simulink model "BMS_MainStateMachine_COM_Harness_SIL"  (R2022b)
settings: configuration reference "BMS_Sw_CodeGenConfig" (kept outside this file)
model workspace (MAT data in the model file):
  BATT.Manufacturer = 'Panasonic'
  BATT.Chemistry = 'Lithium Ion'
  BATT.Model = 'UR18650ZTA'
  BATT.Diameter = 18.2399997711
  BATT.Length = 65.0999984741
  BATT.CycleLife = 500
  BATT.Package.Ns_Module = 1
  BATT.Package.NumModules = 3
  BATT.Capacity.Rate = 2.84999990463
  BATT.Capacity.Min = 2.90000009537
  BATT.Capacity.Max = 3.09999990463
  BATT.Capacity.MaxQ = 3.30460000038
  BATT.Capacity.Type = 3
  BATT.Res.R0 = 0.0113329999149
  BATT.Res.R1 = 0.00999999977648
  BATT.Res.C1 = 0.00300000002608
  BATT.Res.R0_EOL = 0.0142999999225
  BATT.Res.lambda = 1.06599998474
  BATT.Voltage.Nominal = 3.70000004768
  BATT.Voltage.NominalVolt = 3.40000009537
  BATT.Voltage.Cut_off = 3
  BATT.Voltage.Init_Dchrg = 3.38000011444
  BATT.Voltage.Full_Dchrg = 4.19999980927
  BATT.Voltage.Max_Chrg = 4.34999990463
  BATT.Voltage.Over = 4.40000009537
  BATT.Voltage.Under = 3
  BATT.Voltage.threshold = 0.5
  BATT.Voltage.V_LUT = [3 3.09999990463 3.20000004768 3.29999995232 3.40000009537 3.5 3.59999990463 3.70000004768 3.79999995232 3.90000009537 4 4.09999990463 4.19999980927]
  BATT.Temperature.Max = 50
  BATT.Temperature.Min = -20
  BATT.Temperature.Nominal = 20
  BATT.Temperature.dQ_dt = 0.00499999988824
  BATT.Temperature.T_LUT = [-20 -15 -10 -5 0 5 10 15 20 25 30 35 40 45 50]
  BATT.Temperature.derate_Fact = [0.598999977112 0.69580000639 0.769999980927 0.824599981308 0.870000004768 0.912999987602 0.949999988079 0.981000006199 1 1.00499999523 1.00999999046 1.01800000668 1.02999997139 1.05700004101 1.10000002384]
  BATT.Current.Dchrg = 6
  BATT.Current.Chrg = 1.45000004768
  BATT.Current.Chrgfast = 2.5
  BATT.Current.ChrgSafe = 0.0579999983311
  BATT.Current.Overthreshold = 0.20000000298
  BATT.Current.threshold = 0.00999999977648
  BATT.Current.CV_Gain = 20
  BATT.SoC.SoC0 = 50
  BATT.SoC.max = 100
  BATT.SoC.min = 0
  BATT.SoC.alpha = 0.25
  BATT.SoC.Values = [0 10 20 30 40 50 60 70 80 90 100]
  BATT.SoC.iter = 10
  BATT.SoC.TableData = [20 30 40 55 70 85 90 100 100 100 100 100 ... (195 elements, 13x15)]
  BATT.Balancing.Mode : BMS_BalMode_Enum (value not decoded)
  BATT.Balancing.ThresholdOn = 0.0250000003725
  BATT.Balancing.ThresholdOff = 0.00999999977648
  BATT.Balancing.BalWaitOff = 5
  BATT.Balancing.BalWaitOn = 10
  BATT.Balancing.Freq = 1000
  BATT.Balancing.Duty = 0.449999988079
  ChrgBit = Simulink.Parameter
  ChrgBit.Value = 0
  ChrgBit.Description = 'charger Fault Bit'
  ChrgBit.DataType = 'uint8'
  ChrgBit.Complexity = 'real'
  ChrgBit.Dimensions = [1 1]
  CntTime = Simulink.Parameter
  CntTime.Value = 500
  CntTime.Description = 'Conector waiting Time'
  CntTime.DataType = 'uint16'
  CntTime.Complexity = 'real'
  CntTime.Dimensions = [1 1]
  CntTimeout = Simulink.Parameter
  CntTimeout.Value = 5000
  CntTimeout.Description = 'Conector Timeout'
  CntTimeout.DataType = 'uint16'
  CntTimeout.Complexity = 'real'
  CntTimeout.Dimensions = [1 1]
  CurrTimeout = Simulink.Parameter
  CurrTimeout.Value = 1000
  CurrTimeout.Description = 'Over Current Timeout'
  CurrTimeout.DataType = 'uint16'
  CurrTimeout.Complexity = 'real'
  CurrTimeout.Dimensions = [1 1]
  FaultResetTime = Simulink.Parameter
  FaultResetTime.Value = 5000
  FaultResetTime.Description = 'Fault Reset waiting Time'
  FaultResetTime.DataType = 'uint16'
  FaultResetTime.Complexity = 'real'
  FaultResetTime.Dimensions = [1 1]
  HighTempBit = Simulink.Parameter
  HighTempBit.Value = 4
  HighTempBit.Description = 'High Temperature Bit'
  HighTempBit.DataType = 'uint8'
  HighTempBit.Complexity = 'real'
  HighTempBit.Dimensions = [1 1]
  InvrBit = Simulink.Parameter
  InvrBit.Value = 1
  InvrBit.Description = 'Inverter Fault Bit'
  InvrBit.DataType = 'uint8'
  InvrBit.Complexity = 'real'
  InvrBit.Dimensions = [1 1]
  LowTempBit = Simulink.Parameter
  LowTempBit.Value = 3
  LowTempBit.Description = 'Low Temperature Bit'
  LowTempBit.DataType = 'uint8'
  LowTempBit.Complexity = 'real'
  LowTempBit.Dimensions = [1 1]
  OverCurrBit = Simulink.Parameter
  OverCurrBit.Value = 2
  OverCurrBit.Description = 'Over Current Bit'
  OverCurrBit.DataType = 'uint8'
  OverCurrBit.Complexity = 'real'
  OverCurrBit.Dimensions = [1 1]
  OverVoltBit = Simulink.Parameter
  OverVoltBit.Value = 6
  OverVoltBit.Description = 'Over voltage Bit'
  OverVoltBit.DataType = 'uint8'
  OverVoltBit.Complexity = 'real'
  OverVoltBit.Dimensions = [1 1]
  Schedule.BMS_CurrentLimitsCalc_Task = 0.1
  Schedule.BMS_MainStateMachine_Task = 0.05
  Schedule.BMS_BalancingLogic_Task = 0.25
  Schedule.BMS_EstimateSOC_Task = 0.2
  Schedule.BMS_EstimateSOH_Task = 0.2
  TempTimeout = Simulink.Parameter
  TempTimeout.Value = 1000
  TempTimeout.Description = 'Teperature Timeout'
  TempTimeout.DataType = 'uint16'
  TempTimeout.Complexity = 'real'
  TempTimeout.Dimensions = [1 1]
  UnderVoltBit = Simulink.Parameter
  UnderVoltBit.Value = 5
  UnderVoltBit.Description = 'Under voltage Bit'
  UnderVoltBit.DataType = 'uint8'
  UnderVoltBit.Complexity = 'real'
  UnderVoltBit.Dimensions = [1 1]
  VoltSensBit = Simulink.Parameter
  VoltSensBit.Value = 7
  VoltSensBit.Description = 'Voltage sensing Bit'
  VoltSensBit.DataType = 'uint8'
  VoltSensBit.Complexity = 'real'
  VoltSensBit.Dimensions = [1 1]
undefined symbols (not defined in the file): BMS_State_Enum
libraries: pil_lib x1
settings Model: DataDictionary=BMS_Arch_DD.sldd  Creator=MAAM  LastModifiedBy=MAAM
settings ConfigSetRef: SourceName=BMS_Sw_CodeGenConfig

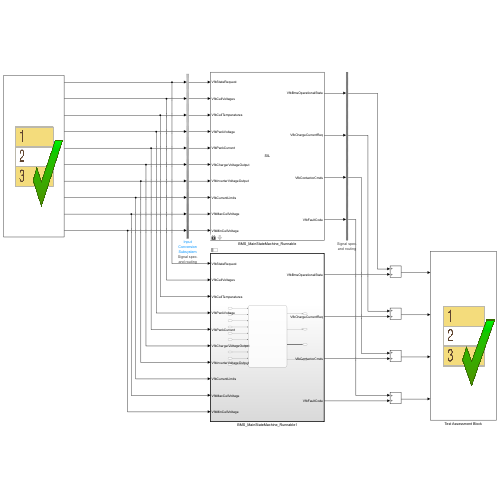
[thumbnail: Simulink's stored preview of the top-level diagram]
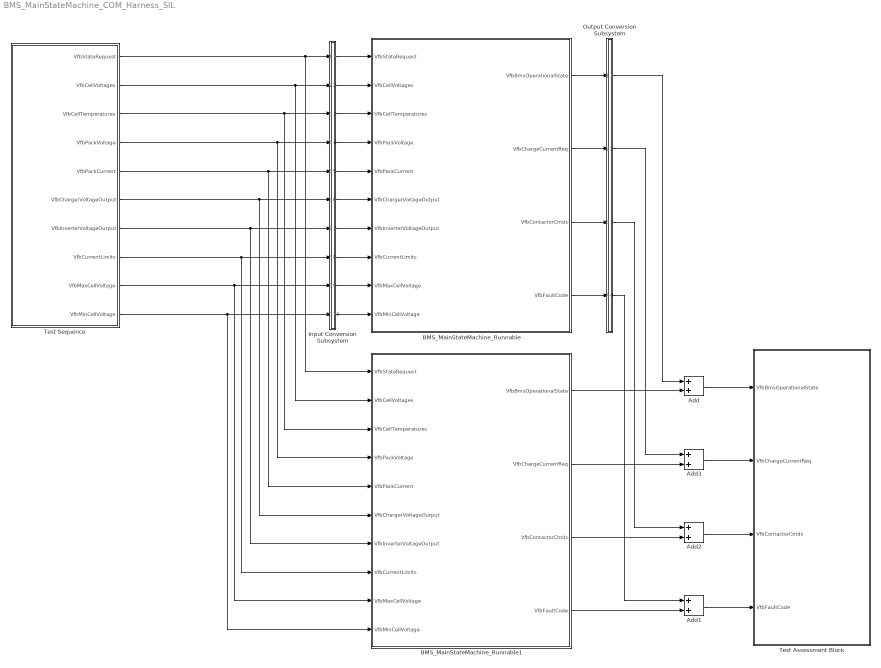
== system BMS_MainStateMachine_COM_Harness_SIL ==
  Add{,1..3} (4 alike) : Sum
  BMS_MainStateMachine_Runnable : Subsystem  Tag=__SL_testing_harness_stub_  DialogController=pil_create_dialog  LoadFcn=|
      | try
      |    if ~strcmp(rtw.pil.getPILVersion, '9.13 (R2022b)_15')
      |       set_param(gcb, 'DialogController', '');
      |       set_param(gcb, 'DialogControllerArgs', '');
      |    end
      | catch e
      |       set_param(gcb, 'DialogController', '');
      |       set_param(gcb, 'DialogControllerArgs', '');
      | end
      mask help: PIL:pil:XILBlockMaskDesc
      mask Display: disp('SIL');
  BMS_MainStateMachine_Runnable1 : Subsystem  Tag=BMS_MainStateMachine_Task  Priority=1  TreatAsAtomicUnit=on  ScheduleAs=Periodic partition  PartitionName=BMS_MainStateMachine_Task  SystemSampleTime=Schedule.BMS_MainStateMachine_Task
      settings: RTWSystemCode=Nonreusable function  RTWFcnNameOpts=Use subsystem name  RTWFileNameOpts=Use subsystem name  FunctionInterfaceSpec=Allow arguments (Optimized)
  Input Conversion Subsystem : Subsystem  Tag=__SLT_ICS__  Description=|
      | Signal spec.
      | and routing
      settings: AttributesFormatString=%<Description>
  Output Conversion Subsystem : Subsystem  Tag=__SLT_OCS__  Description=|
      | Signal spec.
      | and routing
      mask init:
      | ICDictionary = get_param(bdroot, 'DataDictionary');
      | if isempty(ICDictionary)
      |    ICScope = Simulink.data.BaseWorkspace;
      | else
      |    ICScope = Simulink.data.DataDictionary(ICDictionary);
      | end
      | 
      | IC3 = Simulink.Bus.createMATLABStruct('BMS_strContactorCmds', [], [1 1], ICScope);
      settings: AttributesFormatString=%<Description>
  Test Assessment Block : Test Sequence  Tag=__SLT_ASMT__  TreatAsAtomicUnit=on
  Test Sequence : Test Sequence  TreatAsAtomicUnit=on
  wires:
  Test Sequence/1(VfbStateRequest) -> BMS_MainStateMachine_Runnable1/1(VfbStateRequest), Input Conversion Subsystem/1(Inport_1)
  Test Sequence/2(VfbCellVoltages) -> BMS_MainStateMachine_Runnable1/2(VfbCellVoltages), Input Conversion Subsystem/2(Inport_2)
  Test Sequence/4(VfbPackVoltage) -> BMS_MainStateMachine_Runnable1/4(VfbPackVoltage), Input Conversion Subsystem/4(Inport_4)
  Test Sequence/5(VfbPackCurrent) -> BMS_MainStateMachine_Runnable1/5(VfbPackCurrent), Input Conversion Subsystem/5(Inport_5)
  Test Sequence/6(VfbChargerVoltageOutput) -> BMS_MainStateMachine_Runnable1/6(VfbChargerVoltageOutput), Input Conversion Subsystem/6(Inport_6)
  Test Sequence/7(VfbInverterVoltageOutput) -> BMS_MainStateMachine_Runnable1/7(VfbInverterVoltageOutput), Input Conversion Subsystem/7(Inport_7)
  Test Sequence/8(VfbCurrentLimits) -> BMS_MainStateMachine_Runnable1/8(VfbCurrentLimits), Input Conversion Subsystem/8(Inport_8)
  Test Sequence/9(VfbMaxCellVoltage) -> BMS_MainStateMachine_Runnable1/9(VfbMaxCellVoltage), Input Conversion Subsystem/9(Inport_9)
  Test Sequence/10(VfbMinCellVoltage) -> BMS_MainStateMachine_Runnable1/10(VfbMinCellVoltage), Input Conversion Subsystem/10(Inport_10)
  Input Conversion Subsystem/1(Outport_1) -> BMS_MainStateMachine_Runnable/1(VfbStateRequest)
  Input Conversion Subsystem/2(Outport_2) -> BMS_MainStateMachine_Runnable/2(VfbCellVoltages)
  Input Conversion Subsystem/3(Outport_3) -> BMS_MainStateMachine_Runnable/3(VfbCellTemperatures)
  Input Conversion Subsystem/4(Outport_4) -> BMS_MainStateMachine_Runnable/4(VfbPackVoltage)
  Input Conversion Subsystem/5(Outport_5) -> BMS_MainStateMachine_Runnable/5(VfbPackCurrent)
  Input Conversion Subsystem/6(Outport_6) -> BMS_MainStateMachine_Runnable/6(VfbChargerVoltageOutput)
  Input Conversion Subsystem/7(Outport_7) -> BMS_MainStateMachine_Runnable/7(VfbInverterVoltageOutput)
  Input Conversion Subsystem/8(Outport_8) -> BMS_MainStateMachine_Runnable/8(VfbCurrentLimits)
  Input Conversion Subsystem/9(Outport_9) -> BMS_MainStateMachine_Runnable/9(VfbMaxCellVoltage)
  Input Conversion Subsystem/10(Outport_10) -> BMS_MainStateMachine_Runnable/10(VfbMinCellVoltage)
  BMS_MainStateMachine_Runnable/1(VfbBmsOperationalState) -> Output Conversion Subsystem/1(Inport_1)
  BMS_MainStateMachine_Runnable/2(VfbChargeCurrentReq) -> Output Conversion Subsystem/2(Inport_2)
  BMS_MainStateMachine_Runnable/3(VfbContactorCmds) -> Output Conversion Subsystem/3(Inport_3)
  BMS_MainStateMachine_Runnable/4(VfbFaultCode) -> Output Conversion Subsystem/4(Inport_4)
  Output Conversion Subsystem/4(Outport_4) -> Add1/1
  Output Conversion Subsystem/3(Outport_3) -> Add2/1
  Output Conversion Subsystem/2(Outport_2) -> Add3/1
  Output Conversion Subsystem/1(Outport_1) -> Add/1
  Test Sequence/3(VfbCellTemperatures) -> BMS_MainStateMachine_Runnable1/3(VfbCellTemperatures), Input Conversion Subsystem/3(Inport_3)
  BMS_MainStateMachine_Runnable1/4(VfbFaultCode) -> Add1/2
  BMS_MainStateMachine_Runnable1/3(VfbContactorCmds) -> Add2/2
  BMS_MainStateMachine_Runnable1/2(VfbChargeCurrentReq) -> Add3/2
  BMS_MainStateMachine_Runnable1/1(VfbBmsOperationalState) -> Add/2
  Add/1 -> Test Assessment Block/1(VfbBmsOperationalState)
  Add3/1 -> Test Assessment Block/2(VfbChargeCurrentReq)
  Add2/1 -> Test Assessment Block/3(VfbContactorCmds)
  Add1/1 -> Test Assessment Block/4(VfbFaultCode)

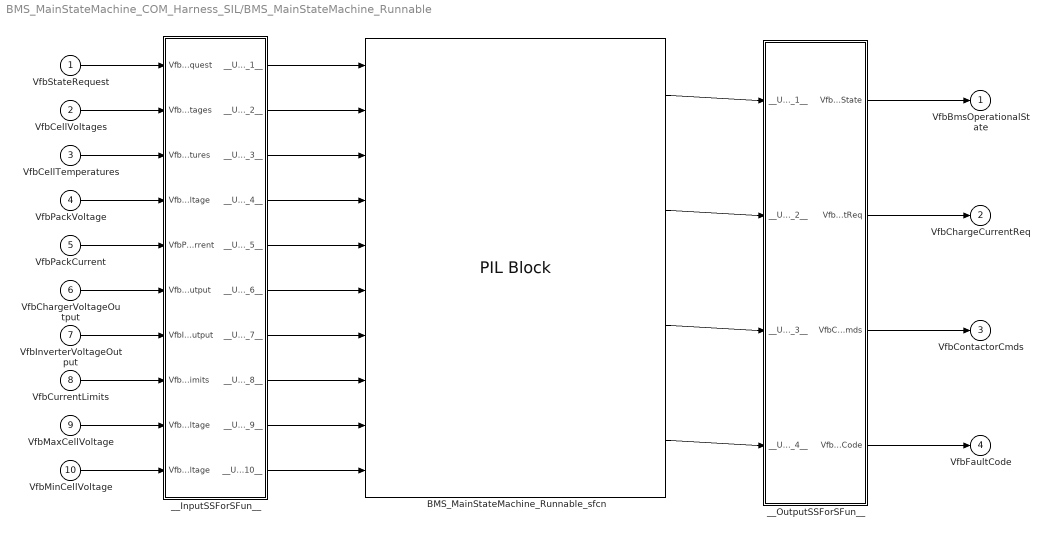
== system BMS_MainStateMachine_COM_Harness_SIL/BMS_MainStateMachine_Runnable ==
  VfbStateRequest : Inport
  VfbCellVoltages : Inport  Port=2  OutDataTypeStr=single  Unit=V  PortDimensions=BATT.Package.NumModules
  VfbCellTemperatures : Inport  Port=3  OutDataTypeStr=single  Unit=°C  PortDimensions=BATT.Package.NumModules
  VfbPackVoltage : Inport  Port=4  OutDataTypeStr=single  Unit=V  PortDimensions=1
  VfbPackCurrent : Inport  Port=5  OutDataTypeStr=single  Unit=A  PortDimensions=1
  VfbChargerVoltageOutput : Inport  Port=6  OutDataTypeStr=single  Unit=V  PortDimensions=1
  VfbInverterVoltageOutput : Inport  Port=7  OutDataTypeStr=single  Unit=V  PortDimensions=1
  VfbCurrentLimits : Inport  Port=8  OutDataTypeStr=single  Unit=A
  VfbMaxCellVoltage : Inport  Port=9  OutDataTypeStr=single  Unit=V  PortDimensions=1
  VfbMinCellVoltage : Inport  Port=10  OutDataTypeStr=single  Unit=V  PortDimensions=1
  BMS_MainStateMachine_Runnable_sfcn : pil_lib/PIL Block  SimulationMode=SIL  IsTopModelPIL=off  CodeDir=BMS_MainStateMachine_Runnable_ert_rtw  AnchorDir=H:\0\New MAAM\10 - MBD\Battary Management System  ConfigName=Software-in-the-Loop (SIL)  XrelIsTopModelCode=on  XrelIsReusable=off  XrelDWorkNames={}  XrelDWorkTypes={}  XrelModelArgVals={}  XrelOrderedParamNames={}
  __InputSSForSFun__ : Subsystem
  __OutputSSForSFun__ : Subsystem
  VfbBmsOperationalState : Outport
  VfbChargeCurrentReq : Outport  Port=2
  VfbContactorCmds : Outport  Port=3  OutDataTypeStr=Bus: BMS_strContactorCmds  SampleTime=[0.050000000000000003 0]  BusOutputAsStruct=on
  VfbFaultCode : Outport  Port=4  OutDataTypeStr=uint8  PortDimensions=1
  wires:
  __OutputSSForSFun__/4(VfbFaultCode) -> VfbFaultCode/1
  __OutputSSForSFun__/3(VfbContactorCmds) -> VfbContactorCmds/1
  __OutputSSForSFun__/2(VfbChargeCurrentReq) -> VfbChargeCurrentReq/1
  __OutputSSForSFun__/1(VfbBmsOperationalState) -> VfbBmsOperationalState/1
  BMS_MainStateMachine_Runnable_sfcn/4 -> __OutputSSForSFun__/4(__UniqueInportName__4__)
  BMS_MainStateMachine_Runnable_sfcn/3 -> __OutputSSForSFun__/3(__UniqueInportName__3__)
  BMS_MainStateMachine_Runnable_sfcn/2 -> __OutputSSForSFun__/2(__UniqueInportName__2__)
  BMS_MainStateMachine_Runnable_sfcn/1 -> __OutputSSForSFun__/1(__UniqueInportName__1__)
  __InputSSForSFun__/10(__UniqueOutportName__10__) -> BMS_MainStateMachine_Runnable_sfcn/10
  __InputSSForSFun__/9(__UniqueOutportName__9__) -> BMS_MainStateMachine_Runnable_sfcn/9
  __InputSSForSFun__/8(__UniqueOutportName__8__) -> BMS_MainStateMachine_Runnable_sfcn/8
  __InputSSForSFun__/7(__UniqueOutportName__7__) -> BMS_MainStateMachine_Runnable_sfcn/7
  __InputSSForSFun__/6(__UniqueOutportName__6__) -> BMS_MainStateMachine_Runnable_sfcn/6
  __InputSSForSFun__/5(__UniqueOutportName__5__) -> BMS_MainStateMachine_Runnable_sfcn/5
  __InputSSForSFun__/4(__UniqueOutportName__4__) -> BMS_MainStateMachine_Runnable_sfcn/4
  __InputSSForSFun__/3(__UniqueOutportName__3__) -> BMS_MainStateMachine_Runnable_sfcn/3
  __InputSSForSFun__/2(__UniqueOutportName__2__) -> BMS_MainStateMachine_Runnable_sfcn/2
  __InputSSForSFun__/1(__UniqueOutportName__1__) -> BMS_MainStateMachine_Runnable_sfcn/1
  VfbMinCellVoltage/1 -> __InputSSForSFun__/10(VfbMinCellVoltage)
  VfbMaxCellVoltage/1 -> __InputSSForSFun__/9(VfbMaxCellVoltage)
  VfbCurrentLimits/1 -> __InputSSForSFun__/8(VfbCurrentLimits)
  VfbInverterVoltageOutput/1 -> __InputSSForSFun__/7(VfbInverterVoltageOutput)
  VfbChargerVoltageOutput/1 -> __InputSSForSFun__/6(VfbChargerVoltageOutput)
  VfbPackCurrent/1 -> __InputSSForSFun__/5(VfbPackCurrent)
  VfbPackVoltage/1 -> __InputSSForSFun__/4(VfbPackVoltage)
  VfbCellTemperatures/1 -> __InputSSForSFun__/3(VfbCellTemperatures)
  VfbCellVoltages/1 -> __InputSSForSFun__/2(VfbCellVoltages)
  VfbStateRequest/1 -> __InputSSForSFun__/1(VfbStateRequest)

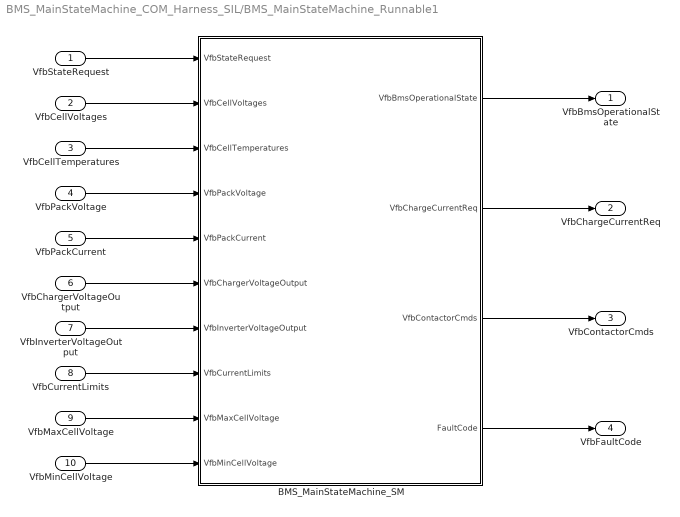
== system BMS_MainStateMachine_COM_Harness_SIL/BMS_MainStateMachine_Runnable1 ==
  VfbStateRequest : Inport
  VfbCellVoltages : Inport  Port=2  OutDataTypeStr=single  Unit=V  PortDimensions=BATT.Package.NumModules
  VfbCellTemperatures : Inport  Port=3  OutDataTypeStr=single  Unit=°C  PortDimensions=BATT.Package.NumModules
  VfbPackVoltage : Inport  Port=4  OutDataTypeStr=single  Unit=V  PortDimensions=1
  VfbPackCurrent : Inport  Port=5  OutDataTypeStr=single  Unit=A  PortDimensions=1
  VfbChargerVoltageOutput : Inport  Port=6  OutDataTypeStr=single  Unit=V  PortDimensions=1
  VfbInverterVoltageOutput : Inport  Port=7  OutDataTypeStr=single  Unit=V  PortDimensions=1
  VfbCurrentLimits : Inport  Port=8  OutDataTypeStr=single  Unit=A
  VfbMaxCellVoltage : Inport  Port=9  OutDataTypeStr=single  Unit=V  PortDimensions=1
  VfbMinCellVoltage : Inport  Port=10  OutDataTypeStr=single  Unit=V  PortDimensions=1
  BMS_MainStateMachine_SM : Stateflow chart  TreatAsAtomicUnit=on
  VfbBmsOperationalState : Outport
  VfbChargeCurrentReq : Outport  Port=2
  VfbContactorCmds : Outport  Port=3  OutDataTypeStr=Bus: BMS_strContactorCmds  BusOutputAsStruct=on
  VfbFaultCode : Outport  Port=4  OutDataTypeStr=uint8  PortDimensions=1
  wires:
  BMS_MainStateMachine_SM/4(FaultCode) -> VfbFaultCode/1
  BMS_MainStateMachine_SM/3(VfbContactorCmds) -> VfbContactorCmds/1
  BMS_MainStateMachine_SM/1(VfbBmsOperationalState) -> VfbBmsOperationalState/1
  VfbMaxCellVoltage/1 -> BMS_MainStateMachine_SM/9(VfbMaxCellVoltage)
  VfbMinCellVoltage/1 -> BMS_MainStateMachine_SM/10(VfbMinCellVoltage)
  BMS_MainStateMachine_SM/2(VfbChargeCurrentReq) -> VfbChargeCurrentReq/1
  VfbCellTemperatures/1 -> BMS_MainStateMachine_SM/3(VfbCellTemperatures)
  VfbInverterVoltageOutput/1 -> BMS_MainStateMachine_SM/7(VfbInverterVoltageOutput)
  VfbPackVoltage/1 -> BMS_MainStateMachine_SM/4(VfbPackVoltage)
  VfbChargerVoltageOutput/1 -> BMS_MainStateMachine_SM/6(VfbChargerVoltageOutput)
  VfbCurrentLimits/1 -> BMS_MainStateMachine_SM/8(VfbCurrentLimits)
  VfbCellVoltages/1 -> BMS_MainStateMachine_SM/2(VfbCellVoltages)
  VfbStateRequest/1 -> BMS_MainStateMachine_SM/1(VfbStateRequest)
  VfbPackCurrent/1 -> BMS_MainStateMachine_SM/5(VfbPackCurrent)

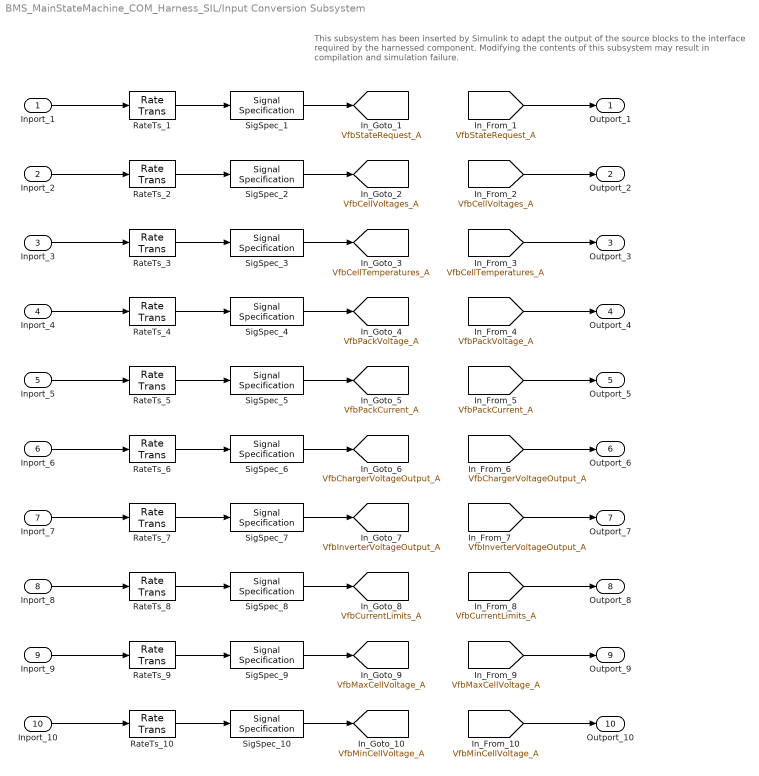
== system BMS_MainStateMachine_COM_Harness_SIL/Input Conversion Subsystem ==
  note: This subsystem has been inserted by Simulink to adapt the output of the source blocks to the interface required by the harnessed component.
      |  Modifying the contents of this subsystem may result in compilation and simulation failure.
  Inport_1 : Inport
  Inport_2 : Inport  Port=2
  Inport_3 : Inport  Port=3
  Inport_4 : Inport  Port=4
  Inport_5 : Inport  Port=5
  Inport_6 : Inport  Port=6
  Inport_7 : Inport  Port=7
  Inport_8 : Inport  Port=8
  Inport_9 : Inport  Port=9
  Inport_10 : Inport  Port=10
  RateTs_1 : RateTransition  InitialCondition=BMS_State_Enum.BMS_Standby  OutPortSampleTime=0.05
  RateTs_{2..10} (9 alike) : RateTransition  OutPortSampleTime=0.05
  SigSpec_1 : SignalSpecification  OutDataTypeStr=Enum: BMS_State_Enum  Dimensions=[1]  SampleTime=0.05
  SigSpec_{4,6..7,9..10} (5 alike) : SignalSpecification  OutDataTypeStr=single  Unit=V  Dimensions=[1]  SampleTime=0.05
  SigSpec_2 : SignalSpecification  OutDataTypeStr=single  Unit=V  Dimensions=[3]  SampleTime=0.05
  SigSpec_3 : SignalSpecification  OutDataTypeStr=single  Unit=°C  Dimensions=[3]  SampleTime=0.05
  SigSpec_5 : SignalSpecification  OutDataTypeStr=single  Unit=A  Dimensions=[1]  SampleTime=0.05
  SigSpec_8 : SignalSpecification  OutDataTypeStr=single  Unit=A  Dimensions=[2]  SampleTime=0.05
  Outport_1 : Outport
  Outport_2 : Outport  Port=2
  Outport_3 : Outport  Port=3
  Outport_4 : Outport  Port=4
  Outport_5 : Outport  Port=5
  Outport_6 : Outport  Port=6
  Outport_7 : Outport  Port=7
  Outport_8 : Outport  Port=8
  Outport_9 : Outport  Port=9
  Outport_10 : Outport  Port=10
  tag scope: VfbCellTemperatures_A=global, VfbCellVoltages_A=global, VfbChargerVoltageOutput_A=global, VfbCurrentLimits_A=global, VfbInverterVoltageOutput_A=global, VfbMaxCellVoltage_A=global, VfbMinCellVoltage_A=global, VfbPackCurrent_A=global, VfbPackVoltage_A=global, VfbStateRequest_A=global
  wires:
  [VfbStateRequest_A] -> Outport_1/1
  SigSpec_1/1 -> [VfbStateRequest_A]
  RateTs_1/1 -> SigSpec_1/1
  Inport_1/1 -> RateTs_1/1
  [VfbCellVoltages_A] -> Outport_2/1
  SigSpec_2/1 -> [VfbCellVoltages_A]
  RateTs_2/1 -> SigSpec_2/1
  Inport_2/1 -> RateTs_2/1
  [VfbCellTemperatures_A] -> Outport_3/1
  SigSpec_3/1 -> [VfbCellTemperatures_A]
  RateTs_3/1 -> SigSpec_3/1
  Inport_3/1 -> RateTs_3/1
  [VfbPackVoltage_A] -> Outport_4/1
  SigSpec_4/1 -> [VfbPackVoltage_A]
  RateTs_4/1 -> SigSpec_4/1
  Inport_4/1 -> RateTs_4/1
  [VfbPackCurrent_A] -> Outport_5/1
  SigSpec_5/1 -> [VfbPackCurrent_A]
  RateTs_5/1 -> SigSpec_5/1
  Inport_5/1 -> RateTs_5/1
  [VfbChargerVoltageOutput_A] -> Outport_6/1
  SigSpec_6/1 -> [VfbChargerVoltageOutput_A]
  RateTs_6/1 -> SigSpec_6/1
  Inport_6/1 -> RateTs_6/1
  [VfbInverterVoltageOutput_A] -> Outport_7/1
  SigSpec_7/1 -> [VfbInverterVoltageOutput_A]
  RateTs_7/1 -> SigSpec_7/1
  Inport_7/1 -> RateTs_7/1
  [VfbCurrentLimits_A] -> Outport_8/1
  SigSpec_8/1 -> [VfbCurrentLimits_A]
  RateTs_8/1 -> SigSpec_8/1
  Inport_8/1 -> RateTs_8/1
  [VfbMaxCellVoltage_A] -> Outport_9/1
  SigSpec_9/1 -> [VfbMaxCellVoltage_A]
  RateTs_9/1 -> SigSpec_9/1
  Inport_9/1 -> RateTs_9/1
  [VfbMinCellVoltage_A] -> Outport_10/1
  SigSpec_10/1 -> [VfbMinCellVoltage_A]
  RateTs_10/1 -> SigSpec_10/1
  Inport_10/1 -> RateTs_10/1

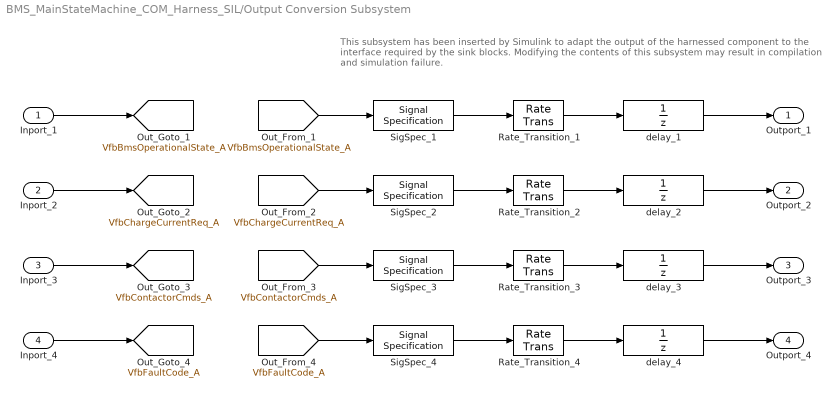
== system BMS_MainStateMachine_COM_Harness_SIL/Output Conversion Subsystem ==
  note: This subsystem has been inserted by Simulink to adapt the output of the harnessed component to the interface required by the sink blocks.
      |  Modifying the contents of this subsystem may result in compilation and simulation failure.
  Inport_1 : Inport
  Inport_2 : Inport  Port=2
  Inport_3 : Inport  Port=3
  Inport_4 : Inport  Port=4
  Rate_Transition_1 : RateTransition  InitialCondition=BMS_State_Enum.BMS_Standby  OutPortSampleTimeOpt=Inherit
  Rate_Transition_2 : RateTransition  OutPortSampleTimeOpt=Inherit
  Rate_Transition_3 : RateTransition  OutPortSampleTimeOpt=Inherit
  Rate_Transition_4 : RateTransition  OutPortSampleTimeOpt=Inherit
  SigSpec_1 : SignalSpecification  OutDataTypeStr=Enum: BMS_State_Enum  Dimensions=[1]  SampleTime=0.05
  SigSpec_2 : SignalSpecification  OutDataTypeStr=single  Unit=A  Dimensions=[1]  SampleTime=0.05
  SigSpec_3 : SignalSpecification  OutDataTypeStr=Bus: BMS_strContactorCmds  Dimensions=[1]  SampleTime=0.05  BusOutputAsStruct=on
  SigSpec_4 : SignalSpecification  OutDataTypeStr=uint8  Dimensions=[1]  SampleTime=0.05
  delay_1 : UnitDelay  InitialCondition=BMS_State_Enum.BMS_Standby  SampleTime=-1
  delay_2 : UnitDelay  SampleTime=-1
  delay_3 : UnitDelay  InitialCondition=IC3  SampleTime=-1
  delay_4 : UnitDelay  SampleTime=-1
  Outport_1 : Outport
  Outport_2 : Outport  Port=2
  Outport_3 : Outport  Port=3
  Outport_4 : Outport  Port=4
  tag scope: VfbBmsOperationalState_A=global, VfbChargeCurrentReq_A=global, VfbContactorCmds_A=global, VfbFaultCode_A=global
  wires:
  Inport_1/1 -> [VfbBmsOperationalState_A]
  [VfbBmsOperationalState_A] -> SigSpec_1/1
  SigSpec_1/1 -> Rate_Transition_1/1
  Rate_Transition_1/1 -> delay_1/1
  delay_1/1 -> Outport_1/1
  Inport_2/1 -> [VfbChargeCurrentReq_A]
  [VfbChargeCurrentReq_A] -> SigSpec_2/1
  SigSpec_2/1 -> Rate_Transition_2/1
  Rate_Transition_2/1 -> delay_2/1
  delay_2/1 -> Outport_2/1
  Inport_3/1 -> [VfbContactorCmds_A]
  [VfbContactorCmds_A] -> SigSpec_3/1
  SigSpec_3/1 -> Rate_Transition_3/1
  Rate_Transition_3/1 -> delay_3/1
  delay_3/1 -> Outport_3/1
  Inport_4/1 -> [VfbFaultCode_A]
  [VfbFaultCode_A] -> SigSpec_4/1
  SigSpec_4/1 -> Rate_Transition_4/1
  Rate_Transition_4/1 -> delay_4/1
  delay_4/1 -> Outport_4/1

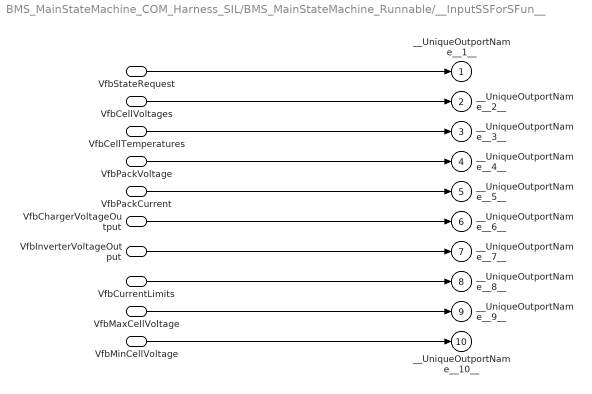
== system BMS_MainStateMachine_COM_Harness_SIL/BMS_MainStateMachine_Runnable/__InputSSForSFun__ ==
  VfbStateRequest : Inport
  VfbCellVoltages : Inport  Port=2  OutDataTypeStr=single  Unit=V  PortDimensions=BATT.Package.NumModules
  VfbCellTemperatures : Inport  Port=3  OutDataTypeStr=single  Unit=°C  PortDimensions=BATT.Package.NumModules
  VfbPackVoltage : Inport  Port=4  OutDataTypeStr=single  Unit=V  PortDimensions=1
  VfbPackCurrent : Inport  Port=5  OutDataTypeStr=single  Unit=A  PortDimensions=1
  VfbChargerVoltageOutput : Inport  Port=6  OutDataTypeStr=single  Unit=V  PortDimensions=1
  VfbInverterVoltageOutput : Inport  Port=7  OutDataTypeStr=single  Unit=V  PortDimensions=1
  VfbCurrentLimits : Inport  Port=8  OutDataTypeStr=single  Unit=A
  VfbMaxCellVoltage : Inport  Port=9  OutDataTypeStr=single  Unit=V  PortDimensions=1
  VfbMinCellVoltage : Inport  Port=10  OutDataTypeStr=single  Unit=V  PortDimensions=1
  __UniqueOutportName__1__ : Outport
  __UniqueOutportName__2__ : Outport  Port=2
  __UniqueOutportName__3__ : Outport  Port=3
  __UniqueOutportName__4__ : Outport  Port=4
  __UniqueOutportName__5__ : Outport  Port=5
  __UniqueOutportName__6__ : Outport  Port=6
  __UniqueOutportName__7__ : Outport  Port=7
  __UniqueOutportName__8__ : Outport  Port=8
  __UniqueOutportName__9__ : Outport  Port=9
  __UniqueOutportName__10__ : Outport  Port=10
  wires:
  VfbMinCellVoltage/1 -> __UniqueOutportName__10__/1
  VfbMaxCellVoltage/1 -> __UniqueOutportName__9__/1
  VfbCurrentLimits/1 -> __UniqueOutportName__8__/1
  VfbInverterVoltageOutput/1 -> __UniqueOutportName__7__/1
  VfbChargerVoltageOutput/1 -> __UniqueOutportName__6__/1
  VfbPackCurrent/1 -> __UniqueOutportName__5__/1
  VfbPackVoltage/1 -> __UniqueOutportName__4__/1
  VfbCellTemperatures/1 -> __UniqueOutportName__3__/1
  VfbCellVoltages/1 -> __UniqueOutportName__2__/1
  VfbStateRequest/1 -> __UniqueOutportName__1__/1

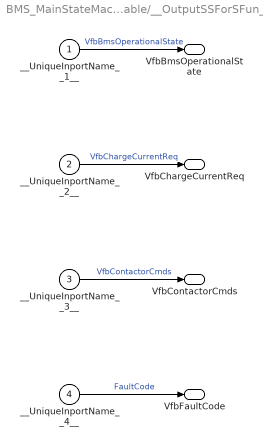
== system BMS_MainStateMachine_COM_Harness_SIL/BMS_MainStateMachine_Runnable/__OutputSSForSFun__ ==
  __UniqueInportName__1__ : Inport
  __UniqueInportName__2__ : Inport  Port=2
  __UniqueInportName__3__ : Inport  Port=3
  __UniqueInportName__4__ : Inport  Port=4
  VfbBmsOperationalState : Outport
  VfbChargeCurrentReq : Outport  Port=2
  VfbContactorCmds : Outport  Port=3  OutDataTypeStr=Bus: BMS_strContactorCmds  SampleTime=[0.050000000000000003 0]  BusOutputAsStruct=on
  VfbFaultCode : Outport  Port=4  OutDataTypeStr=uint8  PortDimensions=1
  wires:
  __UniqueInportName__4__/1 -> VfbFaultCode/1  "FaultCode"
  __UniqueInportName__3__/1 -> VfbContactorCmds/1  "VfbContactorCmds"
  __UniqueInportName__2__/1 -> VfbChargeCurrentReq/1  "VfbChargeCurrentReq"
  __UniqueInportName__1__/1 -> VfbBmsOperationalState/1  "VfbBmsOperationalState"

== stateflow chart BMS_MainStateMachine_COM_Harness_SIL/Test Assessment Block ==
  state Run
    state step_1_1
    state step_1_2
    (default) -> (junction 22)
    Run -> (junction 22)
    (junction 22) -> (junction 23) [order 1] : [t < 5
        | ]
    (junction 23) -> step_1_1 [order 1] : [~in(Run.step_1_1)]
    (junction 23) -> (junction 26) [order 2]
    (junction 31) -> (junction 32)
    (junction 32) -> step_1_2 [order 1] : [~in(Run.step_1_2)]
    (junction 32) -> (junction 35) [order 2]
    (junction 22) -> (junction 31) [order 2]
  (default) -> Run
  data: VfbBmsOperationalState input Enum: BMS_State_Enum size=[1]; VfbChargeCurrentReq input single size=[1]; VfbContactorCmds input Bus: BMS_strContactorCmds size=[1]; VfbFaultCode input uint8 size=[1]

== stateflow chart BMS_MainStateMachine_COM_Harness_SIL/BMS_MainStateMachine_Runnable1/BMS_MainStateMachine_SM ==
  state FaultMonotorig [parallel]
    settings: executionOrder=1
    state FaultReset [parallel]
      settings: executionOrder=1
      state WaitFaultReset
      state ResetFaultCode
        en: FaultCode = uint8(0);
      (default) -> WaitFaultReset
      ResetFaultCode -> WaitFaultReset
      WaitFaultReset -> ResetFaultCode : [VfbStateRequest == BMS_State_Enum.BMS_FaultReset && ...
          |  after(FaultResetTime, msec)]
    state MonitorCurrLim [parallel]
      settings: executionOrder=2
      state NoCurrLimFault
        en:
        FaultCode = bitand(FaultCode, bitcmp(bitshift(uint8(1),OverCurrBit)));
      state OverCurrLimFault
        en:FaultCode = bitor(FaultCode, bitshift(uint8(1),OverCurrBit));
      (default) -> NoCurrLimFault
      OverCurrLimFault -> NoCurrLimFault
      NoCurrLimFault -> OverCurrLimFault [order 2] : [VfbBmsOperationalState == BMS_State_Enum.BMS_Driving && ...
          | duration(((VfbPackCurrent - VfbCurrentLimits(DchargeIndex)) > Current_Overthreshold) ...
          |                                                 > CurrTimeout, msec)]
      NoCurrLimFault -> OverCurrLimFault [order 1] : [VfbBmsOperationalState == BMS_State_Enum.BMS_Charging && ...
          | duration(((VfbPackCurrent - VfbCurrentLimits(ChargeIndex)) > Current_Overthreshold) ...
          |                                                 > CurrTimeout, msec)]
    state MonitorCellTemp [parallel]
      settings: executionOrder=3
      state NoCellTempFault
        en:
        FaultCode = bitand(FaultCode, bitcmp(bitshift(uint8(1),HighTempBit)));
        FaultCode = bitand(FaultCode, bitcmp(bitshift(uint8(1),LowTempBit)));
        en, du:
        MaxCellTemp = max(VfbCellTemperatures);
        MinCellTemp = min(VfbCellTemperatures);
      state HighCellTempFault
        en:FaultCode = bitor(FaultCode, bitshift(uint8(1),HighTempBit));
      state LowCellTempFault
        en:FaultCode = bitor(FaultCode, bitshift(uint8(1),LowTempBit));
      (default) -> FaultMonotorig.MonitorCellTemp.NoCellTempFault
      FaultMonotorig.MonitorCellTemp.NoCellTempFault -> (junction 186) [order 2] : [duration((MinCellTemp < Temperature_Min) > TempTimeout, msec)]
      FaultMonotorig.MonitorCellTemp.NoCellTempFault -> (junction 188) [order 1] : [duration((MaxCellTemp > Temperature_Max) > TempTimeout, msec)]
      (junction 188) -> HighCellTempFault
      (junction 186) -> LowCellTempFault
    state MonitorCellVoltage [parallel]
      settings: executionOrder=4
      state NoCellTempFault
        en:
        FaultCode = bitand(FaultCode, bitcmp(bitshift(uint8(1),OverVoltBit)));
        FaultCode = bitand(FaultCode, bitcmp(bitshift(uint8(1),UnderVoltBit)));
        FaultCode = bitand(FaultCode, bitcmp(bitshift(uint8(1),VoltSensBit)));
        en, du:
        VoltDelta = abs(VfbPackVoltage - sum(VfbCellVoltages))
      state VoltSensFault
        en:FaultCode = bitor(FaultCode, bitshift(uint8(1),VoltSensBit));
      state UnderCellVoltFault
        en:FaultCode = bitor(FaultCode, bitshift(uint8(1),UnderVoltBit));
      state OverCellVoltFault
        en:FaultCode = bitor(FaultCode, bitshift(uint8(1),OverVoltBit));
      (default) -> FaultMonotorig.MonitorCellVoltage.NoCellTempFault
      FaultMonotorig.MonitorCellVoltage.NoCellTempFault -> (junction 203) [order 1] : [VfbMaxCellVoltage >= Voltage_Over]
      (junction 203) -> (junction 210)
      FaultMonotorig.MonitorCellVoltage.NoCellTempFault -> (junction 204) [order 2] : [VfbMinCellVoltage <= Voltage_Under]
      (junction 204) -> (junction 213)
      FaultMonotorig.MonitorCellVoltage.NoCellTempFault -> (junction 216) [order 3] : [VoltDelta > Voltage_threshold]
      (junction 216) -> (junction 218)
      (junction 218) -> VoltSensFault
      (junction 213) -> UnderCellVoltFault
      (junction 210) -> OverCellVoltFault
  state InverterCotactorCmd [parallel]
    settings: executionOrder=2
    state CloseInverter
      state CloseNegInverterRelay
        en: VfbContactorCmds.InverterNegativePole = true;
      state ClosePreInverterRelay
        en: VfbContactorCmds.InverterPreCharge = true;
      state ClosePosInverterRelay
        en: VfbContactorCmds.InverterPositivePole = true;
      state OpenPreInverterRelay
        en: VfbContactorCmds.InverterPreCharge = false;
        InvrCntState = BMS_Conector_Enum.CNT_Close;
      state OpenPosInverterRelay
        en: FaultCode = bitor(FaultCode, bitshift(uint8(1),InvrBit));
      (default) -> CloseNegInverterRelay : {InvrCntState = BMS_Conector_Enum.CNT_Init;}
      CloseNegInverterRelay -> InverterCotactorCmd.CloseInverter.ClosePreInverterRelay : after(CntTime, msec)
      InverterCotactorCmd.CloseInverter.ClosePreInverterRelay -> (junction 147) [order 2] : after(CntTimeout, msec)
      (junction 147) -> (junction 151)
      InverterCotactorCmd.CloseInverter.ClosePreInverterRelay -> ClosePosInverterRelay [order 1] : [VfbInverterVoltageOutput >= VfbPackVoltage]
      ClosePosInverterRelay -> InverterCotactorCmd.CloseInverter.OpenPreInverterRelay : after(CntTime, msec)
      (junction 151) -> InverterCotactorCmd.CloseInverter.OpenPosInverterRelay
    state OpenInverter
      state ClosePreInverterRelay
        en: VfbContactorCmds.InverterPreCharge = true;
      state OpenPosInverterRelay
        en: VfbContactorCmds.InverterPositivePole = false;
      state OpenPreInverterRelay
        en: VfbContactorCmds.InverterPreCharge = false;
      state OpenNegInverterRelay
        en: VfbContactorCmds.InverterNegativePole = false;
        InvrCntState = BMS_Conector_Enum.CNT_Open;
        FaultCode = bitand(FaultCode, bitcmp(bitshift(uint8(1),InvrBit)));
      (default) -> InverterCotactorCmd.OpenInverter.ClosePreInverterRelay : {InvrCntState = BMS_Conector_Enum.CNT_Init;}
      InverterCotactorCmd.OpenInverter.ClosePreInverterRelay -> InverterCotactorCmd.OpenInverter.OpenPosInverterRelay : after(CntTime, msec)
      InverterCotactorCmd.OpenInverter.OpenPosInverterRelay -> InverterCotactorCmd.OpenInverter.OpenPreInverterRelay : after(CntTime, msec)
      InverterCotactorCmd.OpenInverter.OpenPreInverterRelay -> OpenNegInverterRelay : after(CntTime, msec)
    (default) -> OpenInverter : {InvrCntState = BMS_Conector_Enum.CNT_Init;
        |  FaultCode = bitand(FaultCode, bitcmp(bitshift(uint8(1),InvrBit)));}
    OpenInverter -> CloseInverter : [~FaultCode && ...
        | VfbStateRequest == BMS_State_Enum.BMS_Driving && ...
        | ChrgCntState == BMS_Conector_Enum.CNT_Open]
    CloseInverter -> OpenInverter : [FaultCode || ...
        | VfbStateRequest ~= BMS_State_Enum.BMS_Driving]
  state MainStateMacine [parallel]
    settings: executionOrder=4
    state Standby
      en, du: VfbBmsOperationalState = BMS_State_Enum.BMS_Standby;
    state Balancing
      en, du: VfbBmsOperationalState = BMS_State_Enum.BMS_Balancing;
    state BMS_Fault
      en, du: VfbBmsOperationalState = BMS_State_Enum.BMS_Fault;
    state BMS_Driving
      en, du: VfbBmsOperationalState = BMS_State_Enum.BMS_Driving;
    state BMS_Charging
      en, du: VfbBmsOperationalState = BMS_State_Enum.BMS_Charging;
    (default) -> Standby
    (junction 94) -> Standby
    (junction 88) -> (junction 94)
    Balancing -> Standby : [(VfbMaxCellVoltage - VfbMinCellVoltage) >= Balancing_ThresholdOff]
    Standby -> Balancing : [(VfbMaxCellVoltage - VfbMinCellVoltage) >= Balancing_ThresholdOn]
    MainStateMacine -> BMS_Fault [order 1] : [FaultCode]
    BMS_Fault -> (junction 88) : [~FaultCode]
    (junction 86) -> (junction 88)
    MainStateMacine -> BMS_Driving [order 2] : [VfbStateRequest == BMS_State_Enum.BMS_Driving && ...
        |     InvrCntState == BMS_Conector_Enum.CNT_Close]
    BMS_Driving -> (junction 86) : [VfbStateRequest ~= BMS_State_Enum.BMS_Driving && ...
        |     InvrCntState == BMS_Conector_Enum.CNT_Init]
    (junction 89) -> (junction 86)
    MainStateMacine -> BMS_Charging [order 3] : [VfbStateRequest == BMS_State_Enum.BMS_Charging && ...
        |    ChrgCntState == BMS_Conector_Enum.CNT_Close]
    BMS_Charging -> (junction 89) : [VfbStateRequest ~= BMS_State_Enum.BMS_Charging && ...
        |     ChrgCntState == BMS_Conector_Enum.CNT_Init]
  state ChargingCurrent [parallel]
    settings: executionOrder=5
    state Charging_Process
      state Pre_Charge_Mode
        en, du: % Apply trickle charge (~0.05–0.1 C) to safely raise cell voltage
        VfbChargeCurrentReq = Current_ChrgSafe;
      state CC_Mode
        en, du:
        VfbChargeCurrentReq = min(Current_Chrg, VfbCurrentLimits(ChargeIndex));
      state CV_Mode
        en, du:
        ChargeDrop = Current_CV_Gain * (VfbMaxCellVoltage - Voltage_Max_Chrg);
        VfbChargeCurrentReq = min(VfbChargeCurrentReq - ChargeDrop, VfbCurrentLimits(ChargeIndex));
      Pre_Charge_Mode -> CC_Mode : [VfbMaxCellVoltage >= Voltage_NominalVolt]
      CC_Mode -> CV_Mode : [VfbMaxCellVoltage >= Voltage_Full_Dchrg]
    state Init
      en:
      VfbChargeCurrentReq = single(0);
    (default) -> Init
    Init -> Pre_Charge_Mode : [VfbBmsOperationalState == BMS_State_Enum.BMS_Charging]
    CV_Mode -> Init : [VfbChargeCurrentReq <= Current_ChrgSafe]
    Charging_Process -> Init : [VfbBmsOperationalState ~= BMS_State_Enum.BMS_Charging]
  state ChargerCotactorCmd [parallel]
    settings: executionOrder=3
    state CloseCharger
      state CloseNegChargeRelay
        en: VfbContactorCmds.ChargerNegativePole = true;
      state ClosePreChargeRelay
        en: VfbContactorCmds.ChargerPreCharge = true;
      state ClosePosChargeRelay
        en: VfbContactorCmds.ChargerPositivePole = true;
      state OpenPreChargeRelay
        en: VfbContactorCmds.ChargerPreCharge = false;
        ChrgCntState = BMS_Conector_Enum.CNT_Close;
      state OpenPosChargeRelay
        en: FaultCode = bitor(FaultCode, bitshift(uint8(1),ChrgBit));
      (default) -> CloseNegChargeRelay : {ChrgCntState = BMS_Conector_Enum.CNT_Init;}
      CloseNegChargeRelay -> ChargerCotactorCmd.CloseCharger.ClosePreChargeRelay : after(CntTime, msec)
      ChargerCotactorCmd.CloseCharger.ClosePreChargeRelay -> (junction 129) [order 2] : after(CntTimeout, msec)
      (junction 129) -> (junction 132)
      ChargerCotactorCmd.CloseCharger.ClosePreChargeRelay -> ClosePosChargeRelay [order 1] : [VfbChargerVoltageOutput >= VfbPackVoltage]
      ClosePosChargeRelay -> ChargerCotactorCmd.CloseCharger.OpenPreChargeRelay : after(CntTime, msec)
      (junction 132) -> ChargerCotactorCmd.CloseCharger.OpenPosChargeRelay
    state OpenCharger
      state ClosePreChargeRelay
        en: VfbContactorCmds.ChargerPreCharge = true;
      state OpenPosChargeRelay
        en: VfbContactorCmds.ChargerPositivePole = false;
      state OpenPreChargeRelay
        en: VfbContactorCmds.ChargerPreCharge = false;
      state OpenNegChargeRelay
        en: VfbContactorCmds.ChargerNegativePole = false;
        ChrgCntState = BMS_Conector_Enum.CNT_Open;
        FaultCode = bitand(FaultCode, bitcmp(bitshift(uint8(1),ChrgBit)));
      (default) -> ChargerCotactorCmd.OpenCharger.ClosePreChargeRelay : {ChrgCntState = BMS_Conector_Enum.CNT_Init;}
      ChargerCotactorCmd.OpenCharger.ClosePreChargeRelay -> ChargerCotactorCmd.OpenCharger.OpenPosChargeRelay : after(CntTime, msec)
      ChargerCotactorCmd.OpenCharger.OpenPosChargeRelay -> ChargerCotactorCmd.OpenCharger.OpenPreChargeRelay : after(CntTime, msec)
      ChargerCotactorCmd.OpenCharger.OpenPreChargeRelay -> OpenNegChargeRelay : after(CntTime, msec)
    (default) -> OpenCharger : {ChrgCntState = BMS_Conector_Enum.CNT_Init;
        |  FaultCode = bitand(FaultCode, bitcmp(bitshift(uint8(1),ChrgBit)));}
    OpenCharger -> CloseCharger : [~FaultCode && ...
        | VfbStateRequest == BMS_State_Enum.BMS_Charging && ...
        | ChrgCntState == BMS_Conector_Enum.CNT_Open]
    CloseCharger -> OpenCharger : [FaultCode || ...
        | VfbStateRequest ~= BMS_State_Enum.BMS_Charging]
  data: VfbStateRequest input Enum: BMS_State_Enum size=1; VfbCellVoltages input single [0.0..5.0]; VfbCellTemperatures input single [-10..60]; VfbPackVoltage input single size=1 [0..120.0]; VfbPackCurrent input single size=1 [-30..30]; VfbChargerVoltageOutput input single size=1 [-180..180]; VfbInverterVoltageOutput input single size=1 [-180..180]; VfbCurrentLimits input single; VfbMaxCellVoltage input single size=1; VfbMinCellVoltage input single size=1; VfbBmsOperationalState output Enum: BMS_State_Enum size=1; VfbChargeCurrentReq output single size=1; VfbContactorCmds output Bus: BMS_strContactorCmds size=1; FaultCode output uint8 size=1 =uint8(0); ChargeIndex constant uint8 size=1 =2; CntTime constant uint16 size=1 =CntTime; ChrgBit constant uint8 size=1 =ChrgBit; InvrBit constant uint8 size=1 =InvrBit; CntTimeout constant uint16 size=1 =CntTimeout; ChrgCntState local Enum: BMS_Conector_Enum size=1 =BMS_Conector_Enum.CNT_Init; InvrCntState local Enum: BMS_Conector_Enum size=1 =BMS_Conector_Enum.CNT_Init; VoltDelta local single size=1 =single(0); MinCellTemp local single size=1 =single(0); MaxCellTemp local single size=1 =single(0); DchargeIndex constant uint8 size=1 =1; CurrTimeout constant uint16 size=1 =CurrTimeout; FaultResetTime constant uint16 size=1 =FaultResetTime; HighTempBit constant uint8 size=1 =HighTempBit; LowTempBit constant uint8 size=1 =LowTempBit; OverCurrBit constant uint8 size=1 =OverCurrBit; OverVoltBit constant uint8 size=1 =OverVoltBit; TempTimeout constant uint16 size=1 =TempTimeout; UnderVoltBit constant uint8 size=1 =UnderVoltBit; VoltSensBit constant uint8 size=1 =VoltSensBit; ChargeDrop local single size=1 =single(0); Current_Overthreshold constant single size=1 =BATT.Current.Overthreshold; Temperature_Max constant single size=1 =BATT.Temperature.Max; Temperature_Min constant single size=1 =BATT.Temperature.Min; Voltage_Over constant single size=1 =BATT.Voltage.Over; Voltage_Under constant single size=1 =BATT.Voltage.Under; Voltage_threshold constant single size=1 =BATT.Voltage.threshold; Balancing_ThresholdOff constant single size=1 =BATT.Balancing.ThresholdOff; Balancing_ThresholdOn constant single size=1 =BATT.Balancing.ThresholdOn; Current_ChrgSafe constant single size=1 =BATT.Current.ChrgSafe; Current_CV_Gain constant single size=1 =BATT.Current.CV_Gain; Voltage_NominalVolt constant single size=1 =BATT.Voltage.NominalVolt; Voltage_Max_Chrg constant single size=1 =BATT.Voltage.Max_Chrg; Voltage_Full_Dchrg constant single size=1 =BATT.Voltage.Full_Dchrg; Current_Chrg constant single size=1 =BATT.Current.Chrg

== stateflow chart BMS_MainStateMachine_COM_Harness_SIL/Test Sequence ==
  settings: updateMethod=DISCRETE  sampleTime=0.05
  state Run
    %% Initialize data outputs.
    VfbStateRequest = BMS_State_Enum.BMS_Standby;
    VfbCellVoltages = single(zeros(3, 1));
    VfbCellTemperatures = single(zeros(3, 1));
    VfbPackVoltage = single(0);
    VfbPackCurrent = single(0);
    VfbChargerVoltageOutput = single(0);
    VfbInverterVoltageOutput = single(0);
    VfbCurrentLimits = single(zeros(2, 1));
    VfbMaxCellVoltage = single(0);
    VfbMinCellVoltage = single(0);
  (default) -> Run
  data: VfbStateRequest output Enum: BMS_State_Enum size=[1]; VfbCellVoltages output single size=[3]; VfbCellTemperatures output single size=[3]; VfbPackVoltage output single size=[1]; VfbPackCurrent output single size=[1]; VfbChargerVoltageOutput output single size=[1]; VfbInverterVoltageOutput output single size=[1]; VfbCurrentLimits output single size=[2]; VfbMaxCellVoltage output single size=[1]; VfbMinCellVoltage output single size=[1]
